simulink library "uavsim3dlib"  (R2022b)
settings: Solver=VariableStepAuto  StartTime=0.0  StopTime=10.0  RelTol=1e-3
undefined symbols (not defined in the file or in its folder): sim3d
libraries: sim3dcameralib x2, sim3dphyssensorlib x1, sim3dlib x1
settings Model: Creator=The MathWorks, Inc.  LastModifiedBy=Pietro Bruschi
settings SolverCC: AlgebraicLoopSolver=TrustRegion  MaxZcPerStep=1
settings DebuggingCC: UnconnectedInputMsg=warning  UnconnectedOutputMsg=warning  UnconnectedLineMsg=warning  SFMachineParentedDataDiag=warning
settings ModelReferenceCC: EnableRefExpFcnMdlSchedulingChecks=on
settings RTWCC: DLArmComputeVersion=19.05

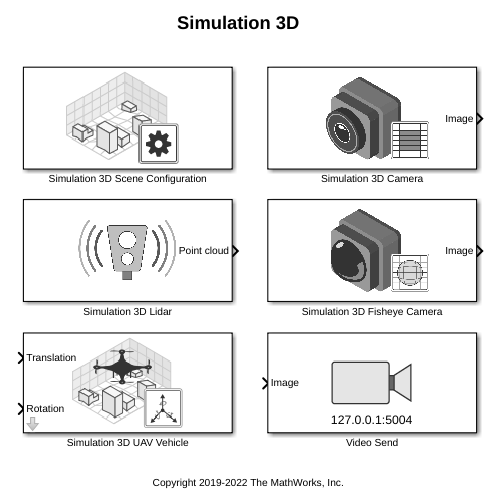
[thumbnail: Simulink's stored preview of the top-level diagram]
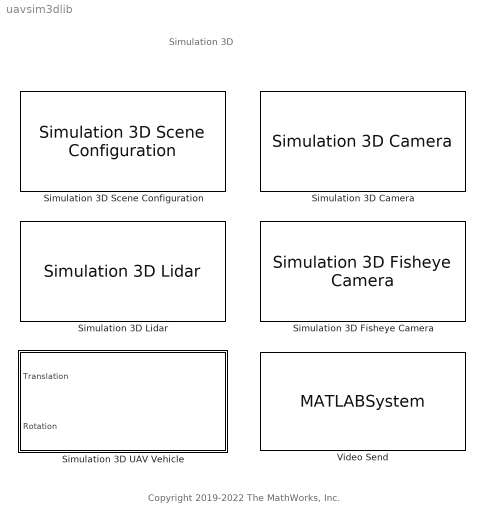
== system uavsim3dlib ==
  note: Simulation 3D
  note: Copyright 2019-2022 The MathWorks, Inc.
  Simulation 3D Camera : sim3dcameralib/Simulation 3D Camera  Priority=1  sensorTag=Sim3dSensor0  sensorId=0  sensorName=Sim3dSensor0  vehTagList={'Scene Origin'}  vehTag=Scene Origin  mountLoc=Origin  offsetFlag=on  tmountOffset=[0, 0, 0]  extTmount=off  rmountOffset=[0, 0, 0]  extRmount=off  FocalLength=[1109, 1109]  OpticalCenter=[640, 360]  ImageSize=[720, 1280]  RadialDistortion=[0, 0]  TangentialDistortion=[0, 0]  SensorSkew=0  DepthOutportEnabled=off  SemanticOutportEnabled=off  TransformOutportEnabled=off  SampleTime=-1  mountPoint=[0 0 0]  mountOrientation=[0 0 0]  aMode=4
  Simulation 3D Fisheye Camera : sim3dcameralib/Simulation 3D Fisheye Camera  Priority=1  sensorTag=Sim3dSensor0  sensorId=0  sensorName=Sim3dSensor0  vehTagList={'Scene Origin'}  vehTag=Scene Origin  mountLoc=Origin  offsetFlag=on  tmountOffset=[0, 0, 0]  extTmount=off  rmountOffset=[0, 0, 0]  extRmount=off  OpticalCenter=[320, 320]  ImageSize=[640, 640]  RadialDistortion=[640, 0, 0, 0]  StretchMatrix=[1, 0; 0, 1]  TransformOutportEnabled=off  SampleTime=-1  mountPoint=[0 0 0]  mountOrientation=[0 0 0]  aMode=4
  Simulation 3D Lidar : sim3dphyssensorlib/Simulation 3D Lidar  Priority=1  sensorTag=Sim3dSensor0  sensorId=0  sensorName=Sim3dSensor0  vehTagList={'Scene Origin'}  vehTag=Scene Origin  mountLoc=Origin  offsetFlag=on  tmountOffset=[0, 0, 0]  rmountOffset=[0, 0, 0]  DetectionRange=120  RangeResolution=0.002  VerticalFOV=40  VerticalResolution=1.25  HorizontalFOV=360  HorizontalResolution=0.16  DistanceOutportEnabled=off  ReflectivityOutportEnabled=off  SemanticOutportEnabled=off  TransformOutportEnabled=off  SampleTime=-1  mountPoint=[0 0 0]  mountOrientation=[0 0 0]  aMode=4
  Simulation 3D Scene Configuration : sim3dlib/Simulation 3D Scene Configuration  Priority=0  ProjectFormat=Default Scenes  SceneDesc=US city block  ProjectName=C:\Program Files\MATLAB\R2022b\toolbox\shared\sim3d_projects\automotive_project\UE4\WindowsNoEditor\VehicleSimulation.exe  ScenePath=/Game/Maps/USCityBlock  EnableOpenDRIVE=off  vehTagList={'Scene Origin'}  vehTag=Scene Origin  OpVisEn=off  Ts=1/60  EnableWindow=on  EnableRemoteAccess=off  EnableWeather=off  SunAltitude=40.0  SunAzimuth=90  clouds=10  wind=1  fog=0  rain=0  EnableGeospatial=off  OriginHeight=200  OriginLatitude=40.744652  OriginLongitude=-73.988864  MapStyle=Aerial  AdditionalAssetIDs=[]  UseAdvancedSunSky=off  SolarTime=11  TimeZone=-5  Day=21  Month=9  Year=2022  UseDaylightSavingTime=on  DSTStartDay=10  DSTStartMonth=3  DSTEndDay=3  DSTEndMonth=11  DSTSwitchHour=2  sensorTag=MainCamera1  sensorId=1  sensorName=MainCamera1  mountLoc=Origin  offsetFlag=off  tmountOffset=[0, 0, 0]  rmountOffset=[0, 0, 0]  HorizontalResolution=1280  VerticalResolution=720  HorizontalFOV=60  mountPoint=[0 0 0]  mountOrientation=[0 0 0]  aMode=4  ID=1  GeoTrigger=Inactive
  Simulation 3D UAV Vehicle : Subsystem  Priority=-1  LoadFcn=sim3d.utils.SimPool.loadCallback(gcb)  mask(Simulation 3D UAV Vehicle){Mesh=Quadrotor, MeshPath=/MathWorksUAVContent/UAVs/HexaRotorUAV/HexaRotor.HexaRotor, Color=Black, ActorName=, InitialTranslation=[0 0 0], InitialRotation=[0 0 0], SampleTime=-1, ActorType=SimulinkVehicle, ID=1, aMode=4, ActorTag=0}
      mask prompts: Mesh "uav:robotsluav:uavvehicle:VehicleType"; MeshPath "uav:robotsluav:uavvehicle:VehicleMeshPath"; Color "uav:robotsluav:uavvehicle:VehicleColor"; ActorName "uav:robotsluav:uavvehicle:VehicleName"; InitialTranslation "uav:robotsluav:uavvehicle:InitialTranslation"; InitialRotation "uav:robotsluav:uavvehicle:InitialRotation"; SampleTime "uav:robotsluav:uavvehicle:SampleTime"
      mask help: uav:robotsluav:uavvehicle:Description
      mask init:
      | uav.sluav.internal.sim3d.UAVVehicleBlockMask.dispatch('maskInitialize', gcb);
      settings: CopyFcn=sim3d.utils.SimPool.copyCallback(gcb)  UndoDeleteFcn=sim3d.utils.SimPool.UndoDeleteCallback(gcb)  PostSaveFcn=sim3d.utils.SimPool.postSaveCallback(gcb)  NameChangeFcn=sim3d.utils.SimPool.nameChangeCallback(gcb)  DestroyFcn=sim3d.utils.SimPool.DestroyCallback(gcb)  PreDeleteFcn=sim3d.utils.SimPool.preDeleteCallback(gcb)
      mask Help: eval('helpview(fullfile(docroot, ''uav'', ''helptargets.map''), ''sim3duavvehicle'')');
      mask TypeOptions Mesh: Simulation 3D UAV/Mesh
      mask Callback Mesh: uav.sluav.internal.sim3d.UAVVehicleBlockMask.dispatch('meshTypeCallback', gcb);
      mask TypeOptions MeshPath: Simulation 3D UAV/MeshPath
      mask TypeOptions Color: Simulation 3D UAV/UAVColor
      mask TypeOptions InitialTranslation: Simulation 3D UAV/Translation
      mask TypeOptions InitialRotation: Simulation 3D UAV/Rotation
      mask TypeOptions SampleTime: Simulation 3D UAV/SampleTime
      mask DialogControl Container4 Prompt: shared_sim3dblks:sim3dblkVehicle:blkDlg_ParameterGroupVar
      mask DialogControl Mesh Prompt: Type:
      mask DialogControl MeshPath Prompt: Path to custom mesh:
      mask DialogControl Color Prompt: Color:
      mask DialogControl ActorName Prompt: Name:
      mask DialogControl Container5 Prompt: shared_sim3dblks:sim3dblkVehicle:blkDlg_Container5
      mask DialogControl InitialTranslation Prompt: Initial Translation (m):
      mask DialogControl InitialRotation Prompt: Initial Rotation (rad):
      mask DialogControl SampleTime Prompt: Sample time:
      mask Display:
      | port_label('input', 1, 'Translation')
      | port_label('input', 2, 'Rotation')
  Video Send : MATLABSystem  System=uav.sluav.internal.system.VideoSend  ImageFormat=RGB  ImageSignal=One multidimensional signal  Compression=JPEG  JPEGQuality=85  VPXFrameDeadline=30  RemoteAddress=127.0.0.1  RemotePort=5004
      mask Type: uav.sluav.internal.system.VideoSend
      mask Display:
      | color('white');
      | plot([100,100,100,100],[100,100,100,100]);
      | plot([0,0,0,0],[0,0,0,0]);
      | image('VideoSend.png','center');
      | color('black');
      | text(50, 15,'\fontsize{12}127.0.0.1:5004','texmode','on','horizontalAlignment', 'center');
      | port_label('input', 1, 'Image');

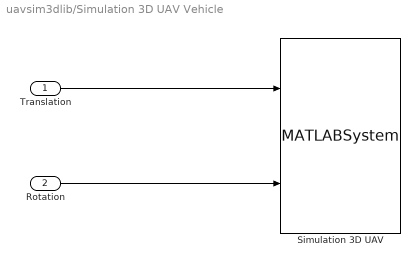
== system uavsim3dlib/Simulation 3D UAV Vehicle ==
  Translation : Inport
  Rotation : Inport  Port=2
  Simulation 3D UAV : MATLABSystem  System=Simulation3DUAV  Translation=InitialTranslation  Rotation=InitialRotation  Mesh=Quadrotor  MeshPath=/MathWorksUAVContent/UAVs/HexaRotorUAV/HexaRotor.HexaRotor  UAVColor=Black  ActorTag=0  SampleTime=SampleTime
      mask Type: Simulation3DUAV
      mask Display:
      | disp('UAV');
      | port_label('input',1,'translation');
      | port_label('input',2,'rotation');
  wires:
  Translation/1 -> Simulation 3D UAV/1
  Rotation/1 -> Simulation 3D UAV/2
